simulink model "single_joint_dynamics_control"  (R2023b)
settings: Solver=FixedStepDiscrete  StartTime=0.0  StopTime=2  FixedStep=0.001  RelTol=1e-3
undefined symbols (not defined in the file or in its folder): DiscIntNeverNeededParam
settings Model: Creator=user  LastModifiedBy=user
settings DebuggingCC: BusObjectLabelMismatch=error
settings HardwareCC: ProdBitPerLong=64  ProdHWDeviceType=Intel->x86-64 (Linux 64)  TargetBitPerLong=64  TargetBitPerPointer=64  TargetBitPerSizeT=64  TargetBitPerPtrDiffT=64  TargetLargestAtomicFloat=Float  TargetIntDivRoundTo=Zero  TargetEndianess=LittleEndian  TargetWordSize=64  TargetHWDeviceType=Intel->x86-64 (Linux 64)  ProdEqTarget=off
settings RTWCC: GenerateReport=on

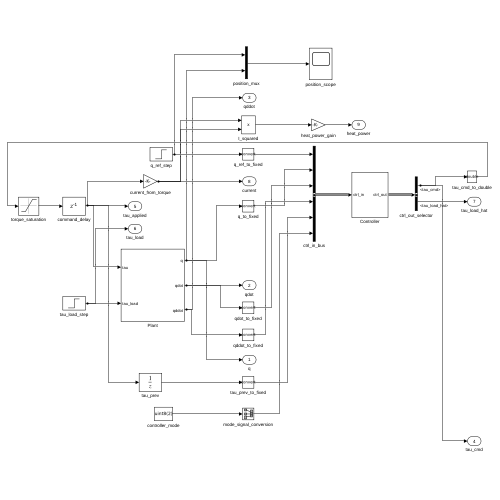
[thumbnail: Simulink's stored preview of the top-level diagram]
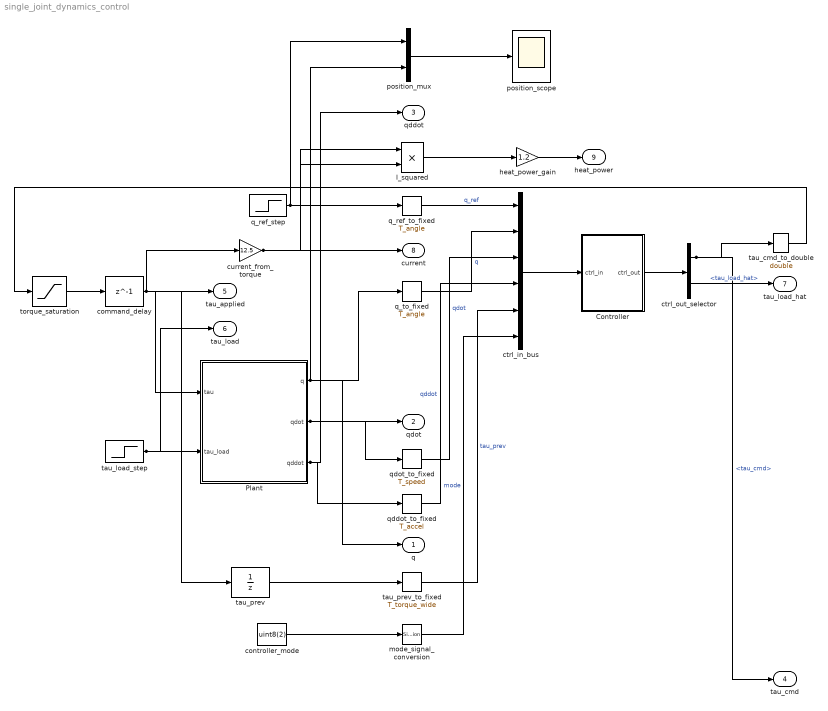
== system single_joint_dynamics_control ==
  Controller : Subsystem  RTWFcnName=usr_pid  RTWFileName=usr_pid
      settings: RTWFcnNameOpts=User specified  RTWFileNameOpts=User specified
  I_squared : Product
  Plant : Subsystem
  command_delay : Delay  DelayLength=1  InitialCondition=0  SampleTime=0.001
  controller_mode : Constant  Value=uint8(2)  OutDataTypeStr=uint8
  ctrl_in_bus : BusCreator  Inputs=6  OutDataTypeStr=Bus: ControllerInputBus
  ctrl_out_selector : BusSelector  OutputSignals=tau_cmd,tau_load_hat
  current_from_torque : Gain  Gain=12.5
  heat_power_gain : Gain  Gain=1.2
  mode_signal_conversion : SignalConversion  OverrideOpt=on
  position_mux : Mux  Inputs=2
  position_scope : Scope
  q_ref_step : Step  Time=0.1  SampleTime=0.001
  q_ref_to_fixed : DataTypeConversion  OutDataTypeStr=T_angle
  q_to_fixed : DataTypeConversion  OutDataTypeStr=T_angle
  qddot_to_fixed : DataTypeConversion  OutDataTypeStr=T_accel
  qdot_to_fixed : DataTypeConversion  OutDataTypeStr=T_speed
  tau_cmd_to_double : DataTypeConversion  OutDataTypeStr=double  SaturateOnIntegerOverflow=off  RndMeth=Floor
  tau_load_step : Step  Time=0.8  After=0.25  SampleTime=0.001
  tau_prev : UnitDelay  SampleTime=0.001  HasFrameUpgradeWarning=on
  tau_prev_to_fixed : DataTypeConversion  OutDataTypeStr=T_torque_wide
  torque_saturation : Saturate  UpperLimit=1.5  LowerLimit=-1.5
  q : Outport
  qdot : Outport  Port=2
  qddot : Outport  Port=3
  tau_cmd : Outport  Port=4
  tau_applied : Outport  Port=5
  tau_load : Outport  Port=6
  tau_load_hat : Outport  Port=7
  current : Outport  Port=8
  heat_power : Outport  Port=9
  wires:
  tau_cmd_to_double/1 -> torque_saturation/1
  ctrl_out_selector/1 -> tau_cmd/1, tau_cmd_to_double/1  "<tau_cmd>"
  Controller/1(ctrl_out) -> ctrl_out_selector/1
  ctrl_in_bus/1 -> Controller/1(ctrl_in)
  mode_signal_conversion/1 -> ctrl_in_bus/6  "mode"
  qdot_to_fixed/1 -> ctrl_in_bus/3  "qdot"
  torque_saturation/1 -> command_delay/1
  command_delay/1 -> tau_prev/1, current_from_torque/1, tau_applied/1, Plant/1(tau)
  qddot_to_fixed/1 -> ctrl_in_bus/4  "qddot"
  tau_prev/1 -> tau_prev_to_fixed/1
  ctrl_out_selector/2 -> tau_load_hat/1  "<tau_load_hat>"
  q_to_fixed/1 -> ctrl_in_bus/2  "q"
  q_ref_step/1 -> position_mux/1, q_ref_to_fixed/1
  heat_power_gain/1 -> heat_power/1
  current_from_torque/1 -> I_squared/1, current/1, I_squared/2
  Plant/1(q) -> q/1, position_mux/2, q_to_fixed/1
  Plant/2(qdot) -> qdot/1, qdot_to_fixed/1
  Plant/3(qddot) -> qddot/1, qddot_to_fixed/1
  tau_load_step/1 -> tau_load/1, Plant/2(tau_load)
  position_mux/1 -> position_scope/1
  tau_prev_to_fixed/1 -> ctrl_in_bus/5  "tau_prev"
  q_ref_to_fixed/1 -> ctrl_in_bus/1  "q_ref"
  controller_mode/1 -> mode_signal_conversion/1
  I_squared/1 -> heat_power_gain/1

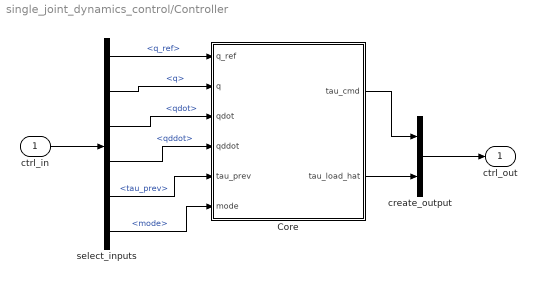
== system single_joint_dynamics_control/Controller ==
  ctrl_in : Inport  OutDataTypeStr=Bus: ControllerInputBus
  Core : MATLAB Function  TreatAsAtomicUnit=on
  create_output : BusCreator  Inputs=2  OutDataTypeStr=Bus: ControllerOutputBus
  select_inputs : BusSelector  OutputSignals=q_ref,q,qdot,qddot,tau_prev,mode
  ctrl_out : Outport  OutDataTypeStr=Bus: ControllerOutputBus
  wires:
  create_output/1 -> ctrl_out/1
  Core/1(tau_cmd) -> create_output/1
  select_inputs/5 -> Core/5(tau_prev)  "<tau_prev>"
  Core/2(tau_load_hat) -> create_output/2
  select_inputs/4 -> Core/4(qddot)  "<qddot>"
  select_inputs/3 -> Core/3(qdot)  "<qdot>"
  select_inputs/2 -> Core/2(q)  "<q>"
  select_inputs/1 -> Core/1(q_ref)  "<q_ref>"
  select_inputs/6 -> Core/6(mode)  "<mode>"
  ctrl_in/1 -> select_inputs/1

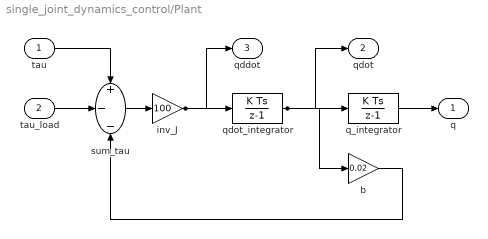
== system single_joint_dynamics_control/Plant ==
  tau : Inport
  tau_load : Inport  Port=2
  b : Gain  Gain=0.02
  inv_J : Gain  Gain=100
  q_integrator : DiscreteIntegrator  gainval=1  SampleTime=0.001  ICPrevOutput=DiscIntNeverNeededParam  ICPrevScaledInput=DiscIntNeverNeededParam
  qdot_integrator : DiscreteIntegrator  gainval=1  SampleTime=0.001  ICPrevOutput=DiscIntNeverNeededParam  ICPrevScaledInput=DiscIntNeverNeededParam
  sum_tau : Sum  Inputs=+--
  q : Outport
  qdot : Outport  Port=2
  qddot : Outport  Port=3
  wires:
  qdot_integrator/1 -> q_integrator/1, qdot/1, b/1
  b/1 -> sum_tau/3
  inv_J/1 -> qddot/1, qdot_integrator/1
  sum_tau/1 -> inv_J/1
  q_integrator/1 -> q/1
  tau_load/1 -> sum_tau/2
  tau/1 -> sum_tau/1

== matlab function single_joint_dynamics_control/Controller/Core ==
  data: q_ref input; tau_cmd output; q input; qdot input; qddot input; tau_prev input; mode input; tau_load_hat output
function [tau_cmd, tau_load_hat] = fcn(q_ref, q, qdot, qddot, tau_prev, mode)
%#codegen
persistent integral_e dob_hat
if isempty(integral_e)
    integral_e = fi(0, 1, 16, 13);
    dob_hat = fi(0, 1, 16, 13);
end
q_ref_f = fi(q_ref, 1, 16, 12);
q_f = fi(q, 1, 16, 12);
qdot_f = fi(qdot, 1, 16, 8);
qddot_f = fi(qddot, 1, 16, 4);
tau_prev_f = fi(tau_prev, 1, 16, 12);
Ts = fi(0.001, 1, 16, 15);
tau_limit = fi(1.5, 1, 16, 13);
integral_limit = fi(0.40000000000000002, 1, 16, 13);
tau_hat_limit = fi(0.80000000000000004, 1, 16, 13);
Kp_pid = fi(8, 1, 16, 10);
Ki_pid = fi(6, 1, 16, 10);
Kd_pid = fi(0.45000000000000001, 1, 16, 14);
Kp_dob = fi(8, 1, 16, 10);
Kd_dob = fi(0.45000000000000001, 1, 16, 14);
Jn_dob = fi(0.01, 1, 16, 15);
bn_dob = fi(0.02, 1, 16, 15);
alpha_dob = fi(0.19741016454517191, 1, 16, 14);
K_imp = fi(4, 1, 16, 10);
D_imp = fi(0.38, 1, 16, 14);
e = fi(q_ref_f - q_f, 1, 16, 12);
tau_cmd = fi(0, 1, 16, 13);
tau_load_hat = fi(0, 1, 16, 13);
if mode < uint8(2)
    integral_e = fi(integral_e + Ts*e, 1, 16, 13);
    if integral_e > integral_limit
        integral_e = integral_limit;
    elseif integral_e < -integral_limit
        integral_e = -integral_limit;
    end
    tau_cmd = fi(Kp_pid*e + Ki_pid*integral_e - Kd_pid*qdot_f, 1, 16, 13);
elseif mode < uint8(3)
    raw_load = fi(tau_prev_f - Jn_dob*qddot_f - bn_dob*qdot_f, 1, 16, 13);
    dob_hat = fi(dob_hat + alpha_dob*(raw_load - dob_hat), 1, 16, 13);
    if dob_hat > tau_hat_limit
        dob_hat = tau_hat_limit;
    elseif dob_hat < -tau_hat_limit
        dob_hat = -tau_hat_limit;
    end
    tau_load_hat = dob_hat;
    tau_cmd = fi(Kp_dob*e - Kd_dob*qdot_f + tau_load_hat, 1, 16, 13);
else
    tau_cmd = fi(K_imp*e - D_imp*qdot_f, 1, 16, 13);
end
if tau_cmd > tau_limit
    tau_cmd = tau_limit;
elseif tau_cmd < -tau_limit
    tau_cmd = -tau_limit;
end
end
